simulink model "Lane_Keeping_Aid"  (R2022b)
settings: Solver=VariableStepAuto  StartTime=0.0  StopTime=10.0  RelTol=1e-3  EnableMultiTasking=on
undefined symbols (not defined in the file): cc_param_150, cc_param_311, cc_param_369, LCFG_DSF_Timeout, LCFG_LKA_Tmr1, LCFG_LKA_Tmr2
settings Model: Creator=rkallum  LastModifiedBy=OTHOMSO1
settings SolverCC: AlgebraicLoopSolver=TrustRegion
settings DataIOCC: LimitDataPoints=on  ReturnWorkspaceOutputs=off
settings OptimizationCC: LifeSpan=inf
settings DebuggingCC: UnconnectedInputMsg=warning  UnconnectedOutputMsg=warning  UnconnectedLineMsg=warning  AllowSymbolicDim=off  SFUnexpectedBacktrackingDiag=warning  SFNoUnconditionalDefaultTransitionDiag=warning  SFExecutionAtInitializationDiag=none  SFMachineParentedDataDiag=warning  UnderSpecifiedDimensionMsg=warning  ArithmeticOperatorsInVariantConditions=warning
settings ModelReferenceCC: EnableRefExpFcnMdlSchedulingChecks=on  PropagateSignalLabelsOutOfModel=off
settings SFSimCC: SimUseLocalCustomCode=off  CustomCodeUndefinedFunction=UseInterfaceOnly
settings RTWCC: RTWUseLocalCustomCode=off
settings CodeAppCC: StateflowObjectComments=on
settings GRTTargetCC: TargetLangStandard=C89/C90 (ANSI)
settings ConfigComp: CovMetricSettings=dw  CovSaveCumulativeToWorkspaceVar=on  CovSaveSingleToWorkspaceVar=on  CovExternalEMLEnable=off

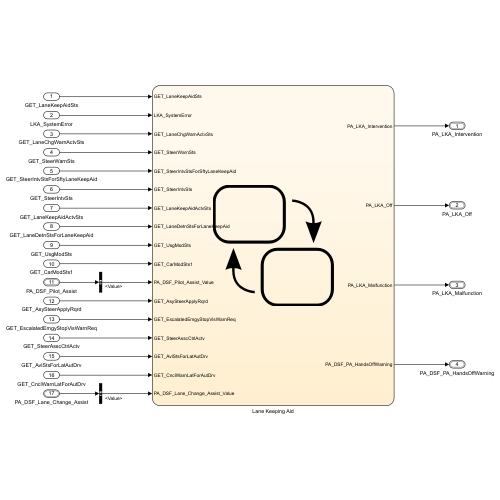
[thumbnail: Simulink's stored preview of the top-level diagram]
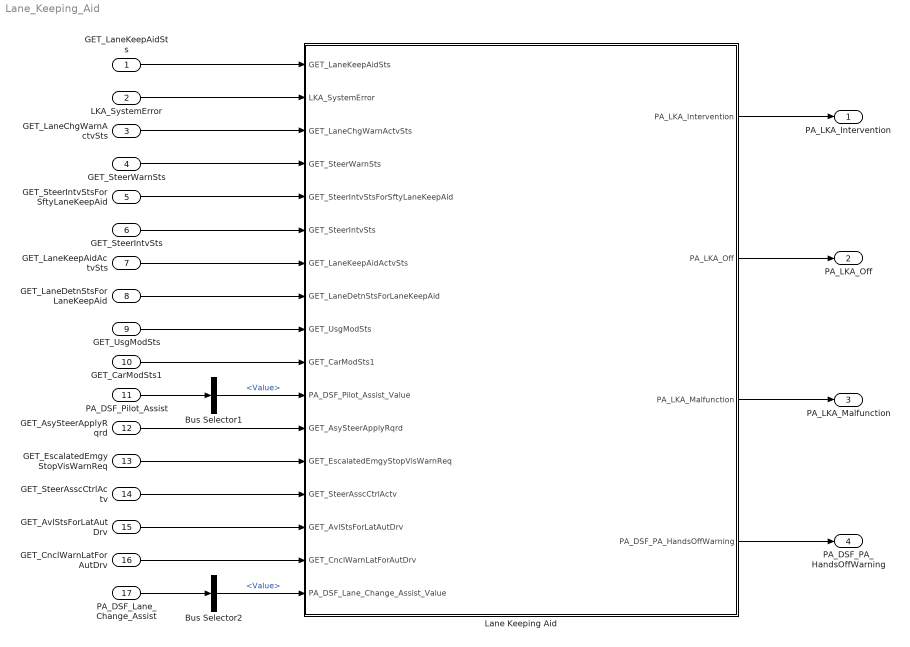
== system Lane_Keeping_Aid ==
  GET_LaneKeepAidSts : Inport  OutDataTypeStr=Enum: FctSts2
  LKA_SystemError : Inport  Port=2  OutDataTypeStr=boolean  SampleTime=0.01
  GET_LaneChgWarnActvSts : Inport  Port=3  OutDataTypeStr=Enum: OnOff1
  GET_SteerWarnSts : Inport  Port=4  OutDataTypeStr=Enum: SteerWarnSts1
  GET_SteerIntvStsForSftyLaneKeepAid : Inport  Port=5  OutDataTypeStr=Enum: SteerIntvSts1
  GET_SteerIntvSts : Inport  Port=6  OutDataTypeStr=Enum: SteerIntvSts1
  GET_LaneKeepAidActvSts : Inport  Port=7  OutDataTypeStr=Enum: OnOff1
  GET_LaneDetnStsForLaneKeepAid : Inport  Port=8  OutDataTypeStr=Enum: LaneDetnSts1
  GET_UsgModSts : Inport  Port=9  OutDataTypeStr=Enum: UsgModSts1
  GET_CarModSts1 : Inport  Port=10  OutDataTypeStr=Enum: CarModSts1
  PA_DSF_Pilot_Assist : Inport  Port=11  OutDataTypeStr=Bus: PA_DSF
  GET_AsySteerApplyRqrd : Inport  Port=12  OutDataTypeStr=Enum: LvlWarn1
  GET_EscalatedEmgyStopVisWarnReq : Inport  Port=13  OutDataTypeStr=Enum: MplLvlVisWarn1
  GET_SteerAsscCtrlActv : Inport  Port=14  OutDataTypeStr=Enum: OnOff1
  GET_AvlStsForLatAutDrv : Inport  Port=15  OutDataTypeStr=Enum: AvlStsForLatAutDrv5
  GET_CnclWarnLatForAutDrv : Inport  Port=16  OutDataTypeStr=Enum: NoYesCrit1
  PA_DSF_Lane_Change_Assist : Inport  Port=17  OutDataTypeStr=Bus: PA_DSF_LCA
  Bus Selector1 : BusSelector  OutputSignals=Value
  Bus Selector2 : BusSelector  OutputSignals=Value
  Lane Keeping Aid : Stateflow chart  TreatAsAtomicUnit=on
      settings: PortSchema="{\"entries\":[{\"content\":{\"sides\":[{\"content\":{\"connectorIds\":[\"In1\",\"In2\",\"In4\",\"In5\",\"In7\",\"In6\",\"In3\",\"In8\",\"In9\",\"In10\",\"In11\",\"In12\",\"In13\",\"In14\",\"In15\",\"In16\",\"In17\"]},\"type\":\"ConnectorPlacement.EquallySpacedRectSide\",\"uuid\":\"81546a12-dbeb-4da3-b971-a88c7786cd62\"},{\"content\":{\"connectorIds\":[\"Out1\",\"Out3\",\"Out4\",\"Out2\"],\"side\":\"RIGHT\"},\"type\":\"ConnectorPlacement.EquallySpacedRectSide\",\"uuid\":\"a13161d3-2edc-41f3-8294-010c24fe0ae7\"},{\"content\":{\"connectorIds\":[],\"side\":\"TOP\"},\"type\":\"ConnectorPlacement.EquallySpacedRectSide\",\"uuid\":\"b219c36a-e050-4b05-acaa-caa7fe0c3a06\"}]},\"type\":\"ConnectorPlacement.EquallySpacedConnector\",\"uuid\":\"81d01f7f-5261-4890-96f8-c0d5b4401501\"}],\"packageUris\":[\"http://schema.mathworks.com/mf0/Connector/R2020b\"],\"version\":\"1.0\"}"
  PA_LKA_Intervention : Outport  OutDataTypeStr=Bus: StatusAndLKAValue
  PA_LKA_Off : Outport  Port=2  OutDataTypeStr=Bus: PA_StatusAndOffOnValue
  PA_LKA_Malfunction : Outport  Port=3  OutDataTypeStr=Bus: PA_StatusAndOffOnValue
  PA_DSF_PA_HandsOffWarning : Outport  Port=4  OutDataTypeStr=Bus: PA_HandsOffWarning
  wires:
  LKA_SystemError/1 -> Lane Keeping Aid/2(LKA_SystemError)
  GET_LaneChgWarnActvSts/1 -> Lane Keeping Aid/4(GET_LaneChgWarnActvSts)
  GET_SteerWarnSts/1 -> Lane Keeping Aid/5(GET_SteerWarnSts)
  GET_SteerIntvStsForSftyLaneKeepAid/1 -> Lane Keeping Aid/7(GET_SteerIntvStsForSftyLaneKeepAid)
  GET_SteerIntvSts/1 -> Lane Keeping Aid/6(GET_SteerIntvSts)
  GET_LaneKeepAidActvSts/1 -> Lane Keeping Aid/3(GET_LaneKeepAidActvSts)
  GET_LaneDetnStsForLaneKeepAid/1 -> Lane Keeping Aid/8(GET_LaneDetnStsForLaneKeepAid)
  Lane Keeping Aid/1(PA_LKA_Intervention) -> PA_LKA_Intervention/1
  GET_UsgModSts/1 -> Lane Keeping Aid/9(GET_UsgModSts)
  GET_CarModSts1/1 -> Lane Keeping Aid/10(GET_CarModSts1)
  PA_DSF_Pilot_Assist/1 -> Bus Selector1/1
  Bus Selector1/1 -> Lane Keeping Aid/11(PA_DSF_Pilot_Assist_Value)  "<Value>"
  Lane Keeping Aid/2(PA_DSF_PA_HandsOffWarning) -> PA_DSF_PA_HandsOffWarning/1
  GET_AsySteerApplyRqrd/1 -> Lane Keeping Aid/12(GET_AsySteerApplyRqrd)
  GET_EscalatedEmgyStopVisWarnReq/1 -> Lane Keeping Aid/13(GET_EscalatedEmgyStopVisWarnReq)
  GET_SteerAsscCtrlActv/1 -> Lane Keeping Aid/14(GET_SteerAsscCtrlActv)
  GET_CnclWarnLatForAutDrv/1 -> Lane Keeping Aid/16(GET_CnclWarnLatForAutDrv)
  GET_AvlStsForLatAutDrv/1 -> Lane Keeping Aid/15(GET_AvlStsForLatAutDrv)
  PA_DSF_Lane_Change_Assist/1 -> Bus Selector2/1
  Bus Selector2/1 -> Lane Keeping Aid/17(PA_DSF_Lane_Change_Assist_Value)  "<Value>"
  Lane Keeping Aid/3(PA_LKA_Off) -> PA_LKA_Off/1
  Lane Keeping Aid/4(PA_LKA_Malfunction) -> PA_LKA_Malfunction/1
  GET_LaneKeepAidSts/1 -> Lane Keeping Aid/1(GET_LaneKeepAidSts)

== stateflow chart Lane_Keeping_Aid/Lane Keeping Aid ==
  state SYSTEM_OK
    state isActive = ActivationCheck [function]
      (default) -> (junction 21)
      (junction 21) -> (junction 22) [order 1] : [GET_CarModSts1==CarModSts1.CarModSts1_CarModNorm &&...
          | GET_UsgModSts==UsgModSts1.UsgModSts1_UsgModDrvg]
      (junction 21) -> (junction 23) [order 2] : {isActive=false;}
      (junction 22) -> (junction 24) : {isActive=true;}
      (junction 24) -> (junction 23)
      (junction 23) -> (junction 25)
    state NOT_ACTIVE
      entry:
      PA_LKA_Intervention.Status = E_CommonStatus.Disabled;
      PA_LKA_Intervention.Value = E_LaneDetection.LKA_No_Lines_Detected;
      PA_DSF_PA_HandsOffWarning.Status = E_CommonStatus.Disabled;
      PA_DSF_PA_HandsOffWarning.Value =  E_HOW_Value.E_HOW_Value_Off;
      PA_LKA_Off.Status = E_CommonStatus.Disabled;
      PA_LKA_Malfunction.Status = E_CommonStatus.Disabled;
      (default) -> (junction 611)
      (junction 611) -> (junction 613) [order 1] : [~LKA_OM]
          | {PA_LKA_Off.Status = E_CommonStatus.NotPresent;
          | PA_LKA_Malfunction.Status = E_CommonStatus.NotPresent;}
      (junction 611) -> (junction 615) [order 2]
      (junction 613) -> (junction 617)
      (junction 617) -> (junction 615)
      (junction 615) -> (junction 620)
    state PENDING_ON
    state PENDING_OFF
    state ACTIVE
      entry:
      PA_LKA_Intervention.Status = E_CommonStatus.Available;
      PA_DSF_PA_HandsOffWarning.Status = E_CommonStatus.Available;
      state activePA = isActivePA [function]
        (default) -> (junction 556)
        (junction 556) -> (junction 557) [order 1] : [PA_DSF_Pilot_Assist_Value==E_DSF_Value.DSF_Active]
        (junction 556) -> (junction 558) [order 2] : {activePA = false;}
        (junction 557) -> (junction 559) : {activePA = true;}
        (junction 559) -> (junction 558)
        (junction 558) -> (junction 560)
      state LKA_ON_OFF [parallel]
        settings: executionOrder=1
        state INVALID_CONFIG
          entry:
          PA_LKA_Off.Status = E_CommonStatus.NotPresent;
        state TT_OFF
          en, du:
          PA_LKA_Off.Status =...
          E_CommonStatus.Available;
          PA_LKA_Off.Value = E_OffOn.Off;
        state TT_ON
          en, du:
          PA_LKA_Off.Value = E_OffOn.On;
        (default) -> (junction 601)
        (junction 601) -> SYSTEM_OK.ACTIVE.LKA_ON_OFF.INVALID_CONFIG [order 2]
        (junction 601) -> SYSTEM_OK.ACTIVE.LKA_ON_OFF.TT_OFF [order 1] : [LKA_OM]
        SYSTEM_OK.ACTIVE.LKA_ON_OFF.TT_OFF -> SYSTEM_OK.ACTIVE.LKA_ON_OFF.TT_ON : %LKA turned Off
            | [GET_LaneKeepAidActvSts==OnOff1.OnOff1_Off]
        SYSTEM_OK.ACTIVE.LKA_ON_OFF.TT_ON -> SYSTEM_OK.ACTIVE.LKA_ON_OFF.TT_OFF : %LKA turned On
            | [GET_LaneKeepAidActvSts==OnOff1.OnOff1_On]
      state LKA_MALFUNCTION [parallel]
        settings: executionOrder=2
        state INVALID_CONFIG
          entry:
          PA_LKA_Malfunction.Status = E_CommonStatus.NotPresent;
        state TT_OFF
          en, du:
          PA_LKA_Malfunction.Status =...
          E_CommonStatus.Available;
          PA_LKA_Malfunction.Value = E_OffOn.Off;
        state TT_ON
          en, du:
          PA_LKA_Malfunction.Value = E_OffOn.On;
        (default) -> (junction 609)
        (junction 609) -> SYSTEM_OK.ACTIVE.LKA_MALFUNCTION.INVALID_CONFIG [order 2]
        (junction 609) -> SYSTEM_OK.ACTIVE.LKA_MALFUNCTION.TT_OFF [order 1] : [LKA_OM]
        SYSTEM_OK.ACTIVE.LKA_MALFUNCTION.TT_OFF -> SYSTEM_OK.ACTIVE.LKA_MALFUNCTION.TT_ON : %LKA system unavailable, telltale to be activated
            | [GET_LaneKeepAidSts==FctSts2.FctSts2_SrvRqrd]
        SYSTEM_OK.ACTIVE.LKA_MALFUNCTION.TT_ON -> SYSTEM_OK.ACTIVE.LKA_MALFUNCTION.TT_OFF : %LKA system available, telltale to be deactivated
            | [GET_LaneKeepAidSts~=FctSts2.FctSts2_SrvRqrd]
      state LKA_INTV [parallel]
        settings: executionOrder=3
        state detLeft = isLineLeft [function]
          (default) -> (junction 421)
          (junction 421) -> (junction 422) [order 1] : [GET_LaneDetnStsForLaneKeepAid==...
              | LaneDetnSts1.LaneDetnSts1_LaneLeDetd ||...
              | GET_LaneDetnStsForLaneKeepAid==...
              | LaneDetnSts1.LaneDetnSts1_LaneLeAndRiDetd]
          (junction 421) -> (junction 423) [order 2] : {detLeft = false;}
          (junction 422) -> (junction 424) : {detLeft = true;}
          (junction 424) -> (junction 423)
          (junction 423) -> (junction 425)
        state detRight = isLineRight [function]
          (default) -> (junction 391)
          (junction 391) -> (junction 392) [order 1] : [GET_LaneDetnStsForLaneKeepAid==...
              | LaneDetnSts1.LaneDetnSts1_LaneRiDetd ||...
              | GET_LaneDetnStsForLaneKeepAid==...
              | LaneDetnSts1.LaneDetnSts1_LaneLeAndRiDetd]
          (junction 391) -> (junction 393) [order 2] : {detRight = false;}
          (junction 392) -> (junction 394) : {detRight = true;}
          (junction 394) -> (junction 393)
          (junction 393) -> (junction 395)
        state intvLeft = isIntvLeft [function]
          (default) -> (junction 351)
          (junction 351) -> (junction 352) [order 1] : [GET_SteerWarnSts==SteerWarnSts1.SteerWarnSts1_WarnOnLeSide ||...
              | GET_SteerIntvSts==SteerIntvSts1.SteerIntvSts1_IntvOnLeSide ||...
              | GET_SteerIntvStsForSftyLaneKeepAid==SteerIntvSts1.SteerIntvSts1_IntvOnLeSide]
          (junction 351) -> (junction 353) [order 2] : {intvLeft = false;}
          (junction 352) -> (junction 354) : {intvLeft = true;}
          (junction 354) -> (junction 353)
          (junction 353) -> (junction 355)
        state intvRight = isIntvRight [function]
          (default) -> (junction 408)
          (junction 408) -> (junction 409) [order 1] : [GET_SteerWarnSts==SteerWarnSts1.SteerWarnSts1_WarnOnRiSide ||...
              | GET_SteerIntvSts==SteerIntvSts1.SteerIntvSts1_IntvOnRiSide ||...
              | GET_SteerIntvStsForSftyLaneKeepAid==SteerIntvSts1.SteerIntvSts1_IntvOnRiSide]
          (junction 408) -> (junction 410) [order 2] : {intvRight = false;}
          (junction 409) -> (junction 411) : {intvRight = true;}
          (junction 411) -> (junction 410)
          (junction 410) -> (junction 412)
        state activeLCA = isActiveLCA [function]
          (default) -> (junction 579)
          (junction 579) -> (junction 580) [order 1] : [PA_DSF_Lane_Change_Assist_Value==E_DSF_LCA.LCA_Executing ||...
              | PA_DSF_Lane_Change_Assist_Value==E_DSF_LCA.LCA_Aborted ||...
              | PA_DSF_Lane_Change_Assist_Value==E_DSF_LCA.LCA_Cancelled]
          (junction 579) -> (junction 581) [order 2] : {activeLCA = false;}
          (junction 580) -> (junction 582) : {activeLCA = true;}
          (junction 582) -> (junction 581)
          (junction 581) -> (junction 583)
        LKA_INTV -> (junction 432)
        (junction 432) -> (junction 369) [order 1] : %China settings
            | [cc_param_369==2]
        (junction 432) -> (junction 366) [order 2]
        (junction 369) -> (junction 385)
        (junction 366) -> (junction 363) [order 1] : %Intervention left with PA active, Argus3, ROW
            | [isIntvLeft && isActivePA && cc_param_311==3]
            | {PA_LKA_Intervention.Value = E_LaneDetection.LKA_Intervention_Left_PA;}
        (junction 385) -> (junction 433) [order 1] : %Intervention left with PA active, Argus3, China
            | [isIntvLeft && isActivePA && cc_param_311==3]
            | {PA_LKA_Intervention.Value = E_LaneDetection.LKA_Intervention_Left_PA_China;}
        (junction 366) -> (junction 386) [order 2]
        (junction 363) -> (junction 388)
        (junction 385) -> (junction 367) [order 2]
        (junction 433) -> (junction 387)
        (junction 386) -> (junction 388) [order 1] : %Intervention right with PA active, Argus3, ROW
            | [isIntvRight && isActivePA && cc_param_311==3]
            | {PA_LKA_Intervention.Value = E_LaneDetection.LKA_Intervention_Right_PA;}
        (junction 367) -> (junction 387) [order 1] : %Intervention right with PA active, Argus3, China
            | [isIntvRight && isActivePA && cc_param_311==3]
            | {PA_LKA_Intervention.Value = E_LaneDetection.LKA_Intervention_Right_PA_China;}
        (junction 386) -> (junction 402) [order 2]
        (junction 388) -> (junction 368)
        (junction 367) -> (junction 403) [order 2]
        (junction 387) -> (junction 404)
        (junction 402) -> (junction 368) [order 1] : %Intervention left/line right detected, Argus3, ROW
            | [isIntvLeft && isLineRight && cc_param_311==3]
            | {PA_LKA_Intervention.Value = E_LaneDetection.LKA_Intv_Left_Det_Right;}
        (junction 403) -> (junction 404) [order 1] : %Intervention left/line right detected, Argus3, China
            | [isIntvLeft && isLineRight && cc_param_311==3]
            | {PA_LKA_Intervention.Value = E_LaneDetection.LKA_Intv_Left_Det_Right_China;}
        (junction 402) -> (junction 370) [order 2]
        (junction 368) -> (junction 362)
        (junction 403) -> (junction 365) [order 2]
        (junction 404) -> (junction 405)
        (junction 370) -> (junction 362) [order 1] : %Intervention right/line left detected, Argus3, ROW
            | [isIntvRight && isLineLeft && cc_param_311==3]
            | {PA_LKA_Intervention.Value = E_LaneDetection.LKA_Intv_Right_Det_Left;}
        (junction 365) -> (junction 405) [order 1] : %Intervention right/line left detected, Argus3, China
            | [isIntvRight && isLineLeft && cc_param_311==3]
            | {PA_LKA_Intervention.Value = E_LaneDetection.LKA_Intv_Right_Det_Left_China;}
        (junction 370) -> (junction 364) [order 2]
        (junction 362) -> (junction 371)
        (junction 365) -> (junction 435) [order 2]
        (junction 405) -> (junction 472)
        (junction 364) -> (junction 371) [order 1] : %Intervention left (line right not detected for Argus3) ROW
            | [isIntvLeft]
            | {PA_LKA_Intervention.Value = E_LaneDetection.LKA_Intervention_Left;}
        (junction 435) -> (junction 472) [order 1] : %Intervention left (line right not detected for Argus3) China
            | [isIntvLeft]
            | {PA_LKA_Intervention.Value = E_LaneDetection.LKA_Intervention_Left_China;}
        (junction 364) -> (junction 440) [order 2]
        (junction 371) -> (junction 439)
        (junction 435) -> (junction 452) [order 2]
        (junction 472) -> (junction 468)
        (junction 440) -> (junction 439) [order 1] : %Intervention right (line left not detected for Argus3) ROW
            | [isIntvRight]
            | {PA_LKA_Intervention.Value = E_LaneDetection.LKA_Intervention_Right;}
        (junction 452) -> (junction 468) [order 1] : %Intervention right (line left not detected for Argus3) China
            | [isIntvRight]
            | {PA_LKA_Intervention.Value = E_LaneDetection.LKA_Intervention_Right_China;}
        (junction 440) -> (junction 475) [order 2]
        (junction 439) -> (junction 436)
        (junction 452) -> (junction 459) [order 2]
        (junction 468) -> (junction 460)
        (junction 436) -> (junction 460)
        (junction 460) -> (junction 447)
        (junction 475) -> (junction 459)
        (junction 459) -> (junction 461) [order 2]
        (junction 461) -> (junction 447) [order 1] : %Show green lines when PA active, Argus3
            | [isActivePA && cc_param_311==3]
            | {PA_LKA_Intervention.Value = E_LaneDetection.LKA_Line_Detected_PA;}
        (junction 459) -> (junction 462) [order 1] : %No lines if no intervention and LKA/PA off or
            | %LCA executing/aborted/cancelled
            | [(GET_LaneKeepAidActvSts==OnOff1.OnOff1_Off &&...
            | GET_LaneChgWarnActvSts==OnOff1.OnOff1_Off &&...
            | ~isActivePA) || isActiveLCA]
            | {PA_LKA_Intervention.Value =...
            | E_LaneDetection.LKA_No_Lines_Detected;}
        (junction 461) -> (junction 453) [order 2]
        (junction 447) -> (junction 469)
        (junction 453) -> (junction 469) [order 1] : %Show grey lines when LKA on and both detected
            | [isLineLeft && isLineRight]
            | {PA_LKA_Intervention.Value = E_LaneDetection.LKA_Line_Detected_Both;}
        (junction 453) -> (junction 457) [order 2]
        (junction 469) -> (junction 458)
        (junction 457) -> (junction 458) [order 1] : %Show grey line when LKA on and left detected
            | [isLineLeft]
            | {PA_LKA_Intervention.Value = E_LaneDetection.LKA_Line_Detected_Left;}
        (junction 457) -> (junction 441) [order 2]
        (junction 458) -> (junction 446)
        (junction 441) -> (junction 446) [order 1] : %Show grey line when LKA on and right detected
            | [isLineRight]
            | {PA_LKA_Intervention.Value = E_LaneDetection.LKA_Line_Detected_Right;}
        (junction 441) -> (junction 454) [order 2] : %Show no lines when LKA on and none detected
            | {PA_LKA_Intervention.Value = E_LaneDetection.LKA_No_Lines_Detected;}
        (junction 446) -> (junction 470)
        (junction 454) -> (junction 462)
        (junction 470) -> (junction 454)
        (junction 462) -> (junction 455)
      state HOW [parallel]
        settings: executionOrder=4
        state HOW_LKA
          state HOW_OFF
            entry:
            PA_DSF_PA_HandsOffWarning.Value =...
            E_HOW_Value.E_HOW_Value_Off;
          state HOW_ON
            entry:
            PA_DSF_PA_HandsOffWarning.Value =...
            E_HOW_Value.E_HOW_Value_Lvl2;
          (default) -> HOW_OFF
          HOW_OFF -> HOW_ON : %HOW requested
              | [hasChangedFrom(GET_AsySteerApplyRqrd, LvlWarn1.LvlWarn1_NoWarn) &&...
              | hasChangedTo(GET_AsySteerApplyRqrd, LvlWarn1.LvlWarn1_Lvl1) ||...
              | hasChangedTo(GET_AsySteerApplyRqrd, LvlWarn1.LvlWarn1_Lvl2)]
          HOW_ON -> HOW_OFF : %HOW not requested
              | [hasChangedTo(GET_AsySteerApplyRqrd, LvlWarn1.LvlWarn1_NoWarn)]
        state HOW_PA
          state OFF
            entry: PA_DSF_PA_HandsOffWarning.Value =...
            E_HOW_Value.E_HOW_Value_Off;
          state Level1
            entry: PA_DSF_PA_HandsOffWarning.Value = E_HOW_Value.E_HOW_Value_Lvl1;
          state Level2
            entry: PA_DSF_PA_HandsOffWarning.Value = E_HOW_Value.E_HOW_Value_Lvl2;
          state Cancel
            entry: PA_DSF_PA_HandsOffWarning.Value = E_HOW_Value.E_HOW_Value_Cancel;
          (default) -> OFF
          OFF -> Level1 [order 1] : %Level 1 warning activated
              | [((hasChangedFrom(GET_AsySteerApplyRqrd, LvlWarn1.LvlWarn1_NoWarn) &&...
              |  hasChangedTo(GET_AsySteerApplyRqrd, LvlWarn1.LvlWarn1_Lvl1))||...
              | (hasChangedFrom(GET_AsySteerApplyRqrd, LvlWarn1.LvlWarn1_Lvl2) &&...
              |  hasChangedTo(GET_AsySteerApplyRqrd, LvlWarn1.LvlWarn1_Lvl1))) &&...
              | GET_SteerAsscCtrlActv == OnOff1.OnOff1_On]
          Level1 -> OFF [order 2] : %Level 1 deactivated due to either No Warning or deactivation of Pilot Assist
              | [(GET_SteerAsscCtrlActv == OnOff1.OnOff1_Off) ||...
              | (hasChangedFrom(GET_AsySteerApplyRqrd, LvlWarn1.LvlWarn1_Lvl1) &&...
              | hasChangedTo(GET_AsySteerApplyRqrd, LvlWarn1.LvlWarn1_NoWarn))]
          Level1 -> Level2 [order 1] : %Level 1 changed to Level 2
              | [(hasChangedFrom(GET_AsySteerApplyRqrd, LvlWarn1.LvlWarn1_Lvl1) &&...
              |  hasChangedTo(GET_AsySteerApplyRqrd, LvlWarn1.LvlWarn1_Lvl2)) &&...
              | GET_SteerAsscCtrlActv == OnOff1.OnOff1_On]
          Level2 -> Level1 [order 1] : %Level 2 changed to Level 1
              | [(hasChangedFrom(GET_AsySteerApplyRqrd, LvlWarn1.LvlWarn1_Lvl2) &&...
              |  hasChangedTo(GET_AsySteerApplyRqrd, LvlWarn1.LvlWarn1_Lvl1)) &&...
              | GET_SteerAsscCtrlActv == OnOff1.OnOff1_On]
          OFF -> Level2 [order 2] : %Level 2 warning activated
              | [((hasChangedFrom(GET_AsySteerApplyRqrd, LvlWarn1.LvlWarn1_NoWarn) &&...
              |  hasChangedTo(GET_AsySteerApplyRqrd, LvlWarn1.LvlWarn1_Lvl2))||...
              | (hasChangedFrom(GET_AsySteerApplyRqrd, LvlWarn1.LvlWarn1_Lvl1) &&...
              |  hasChangedTo(GET_AsySteerApplyRqrd, LvlWarn1.LvlWarn1_Lvl2))) &&...
              | GET_SteerAsscCtrlActv == OnOff1.OnOff1_On]
          Level2 -> OFF [order 2] : %Level 2 deactivated due to either No Warning or deactivation of Pilot Assist
              | [(GET_SteerAsscCtrlActv == OnOff1.OnOff1_Off) ||...
              | (hasChangedFrom(GET_AsySteerApplyRqrd, LvlWarn1.LvlWarn1_Lvl2) &&...
              |  hasChangedTo(GET_AsySteerApplyRqrd, LvlWarn1.LvlWarn1_NoWarn))]
          Level2 -> Cancel [order 3] : %Pilot Assist is deactivated and a "Cancel" message is shown
              | [GET_CnclWarnLatForAutDrv == NoYesCrit1.NoYesCrit1_Yes &&...
              |  GET_AvlStsForLatAutDrv == AvlStsForLatAutDrv5.AvlStsForLatAutDrv5_DrvrNotInLoopDetd]
          Level2 -> Cancel [order 4] : %Escalated Emergency Stop activated and "Cancel" message is shown
              | [GET_EscalatedEmgyStopVisWarnReq==MplLvlVisWarn1.MplLvlVisWarn1_WarnLvl1]
          Cancel -> OFF : %Cancel Message removed
              | [after(LCFG_DSF_Timeout, sec)]
        (default) -> (junction 551)
        (junction 551) -> HOW_LKA [order 2]
        (junction 551) -> HOW_PA [order 1] : [isActivePA]
        HOW_LKA -> HOW_PA : [isActivePA]
        HOW_PA -> HOW_LKA : [~isActivePA]
    (default) -> NOT_ACTIVE
    NOT_ACTIVE -> PENDING_ON : [ActivationCheck()]
    PENDING_ON -> NOT_ACTIVE [order 1] : [~ActivationCheck()]
    PENDING_OFF -> NOT_ACTIVE [order 1] : [after(LCFG_LKA_Tmr1,sec)]
    PENDING_ON -> ACTIVE [order 2] : [after(LCFG_LKA_Tmr2,sec)]
    PENDING_OFF -> ACTIVE [order 2] : [ActivationCheck()]
    ACTIVE -> PENDING_OFF : [~ActivationCheck()]
  state SYSTEM_ERROR
    entry:
    PA_LKA_Intervention.Status = E_CommonStatus.SystemError;
    PA_LKA_Intervention.Value = E_LaneDetection.LKA_No_Lines_Detected;
    PA_DSF_PA_HandsOffWarning.Status = E_CommonStatus.SystemError;
    PA_LKA_Off.Status = E_CommonStatus.SystemError;
    PA_LKA_Malfunction.Status = E_CommonStatus.SystemError;
  (default) -> (junction 192)
  (junction 192) -> (junction 599) [order 2] : {LKA_OM = false;}
  (junction 192) -> (junction 7) [order 1] : % Show LKA off, malf
      | [cc_param_150==3 ||...
      | cc_param_311==3]
      | {LKA_OM = true;}
  (junction 599) -> SYSTEM_OK
  (junction 7) -> SYSTEM_OK [order 2]
  (junction 7) -> (junction 9) [order 1] : [LKA_SystemError==true]
  SYSTEM_OK -> SYSTEM_ERROR : [LKA_SystemError==true]
  SYSTEM_ERROR -> SYSTEM_OK : [LKA_SystemError==false]
  (junction 9) -> SYSTEM_ERROR
  data: isActive function_output boolean; activePA function_output; detLeft function_output; detRight function_output; intvLeft function_output; intvRight function_output; activeLCA function_output; GET_LaneKeepAidSts input Enum: FctSts2; LCFG_LKA_Tmr2 parameter; LCFG_LKA_Tmr1 parameter; LKA_SystemError input boolean; GET_LaneKeepAidActvSts input Enum: OnOff1; GET_LaneChgWarnActvSts input Enum: OnOff1; GET_SteerWarnSts input Enum: SteerWarnSts1; GET_SteerIntvSts input Enum: SteerIntvSts1; GET_SteerIntvStsForSftyLaneKeepAid input Enum: SteerIntvSts1; GET_LaneDetnStsForLaneKeepAid input Enum: LaneDetnSts1; GET_UsgModSts input Enum: UsgModSts1; GET_CarModSts1 input Enum: CarModSts1; cc_param_369 parameter uint8; PA_LKA_Intervention output Bus: StatusAndLKAValue; PA_DSF_Pilot_Assist_Value input; cc_param_150 parameter; PA_DSF_PA_HandsOffWarning output Bus: PA_HandsOffWarning; GET_AsySteerApplyRqrd input Enum: LvlWarn1; GET_EscalatedEmgyStopVisWarnReq input Enum: MplLvlVisWarn1; GET_SteerAsscCtrlActv input Enum: OnOff1; GET_AvlStsForLatAutDrv input Enum: AvlStsForLatAutDrv5; GET_CnclWarnLatForAutDrv input Enum: NoYesCrit1; LCFG_DSF_Timeout parameter; PA_DSF_Lane_Change_Assist_Value input Enum: E_DSF_LCA; PA_LKA_Off output Bus: PA_StatusAndOffOnValue; PA_LKA_Malfunction output Bus: PA_StatusAndOffOnValue; NoLKA local boolean; cc_param_311 parameter; LKA_OM local
